simulink model "punto_33"  (R2015a)
settings: Solver=ode45  StartTime=0.0  StopTime=10.0  RelTol=1e-3
values from neighbouring files (symbols this model uses):
  a = [-6 -11 -6;1 0 0;0 1 0]    [punto_1.m]    (also in punto_2.m = [0 1 0;0 0 1;-5 -6 0]; punto_3.m = [0 1 0;0 0 1;-1.244 -0.3956 -3.145]; punto_4.m = [0 1;0 0])
  Aaux = Abb-Ko*Aab    [punto_3.m]    (also in punto_4.m)
  b = [1;0;0]    [punto_1.m]    (also in punto_2.m = [0;0;1]; punto_3.m = [0;0;1.244]; punto_4.m = [0;1])
  Baux = Aaux*Ko+Aba+Ko*Aaa    [punto_3.m]    (also in punto_4.m)
  c = [0 0 10]    [punto_1.m]    (also in punto_2.m = [1 0 0]; punto_3.m = [1 0 0]; punto_4.m = [1 0])
  d = 0    [punto_1.m]    (also in punto_2.m; punto_3.m; punto_4.m)
  F = Bb-(Ko*Ba)    [punto_3.m]    (also in punto_4.m)
  k = place(a,b,p)    [punto_1.m]    (also in punto_2.m = acker(a,b,p); punto_3.m = place(a,b,p1); punto_4.m = place(a,b,prealim))
  Ko = acker(a',c',p)'    [punto_2.m]    (also in punto_3.m = place(Abb',Aab',p)'; punto_4.m = place(Abb',Aab',pobsv)')
settings Model: Creator=Jose Roldan  LastModifiedBy=Jose Roldan

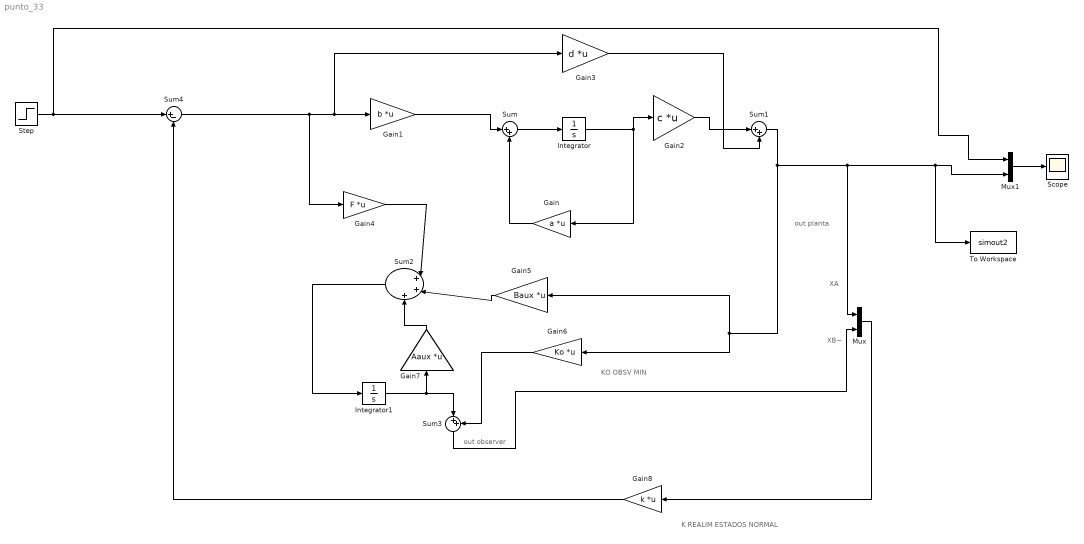
== system punto_33 ==
  note: KO OBSV MIN
  note: K REALIM ESTADOS NORMAL
  note: out planta
  note: out observer
  note: XB~
  note: XA
  Gain : Gain  Gain=a  Multiplication=Matrix(K*u)
  Gain1 : Gain  Gain=b  Multiplication=Matrix(K*u)
  Gain2 : Gain  Gain=c  Multiplication=Matrix(K*u)
  Gain3 : Gain  Gain=d  Multiplication=Matrix(K*u)
  Gain4 : Gain  Gain=F  Multiplication=Matrix(K*u)
  Gain5 : Gain  Gain=Baux  Multiplication=Matrix(K*u)
  Gain6 : Gain  Gain=Ko  Multiplication=Matrix(K*u)
  Gain7 : Gain  Gain=Aaux  Multiplication=Matrix(K*u)
  Gain8 : Gain  Gain=k  Multiplication=Matrix(K*u)
  Integrator : Integrator
  Integrator1 : Integrator
  Mux : Mux  Inputs=2
  Mux1 : Mux  Inputs=2
  Scope : Scope
  Step : Step  SampleTime=0
  Sum : Sum  Inputs=|++
  Sum1 : Sum  Inputs=|++
  Sum2 : Sum  Inputs=|+++
  Sum3 : Sum  Inputs=|++
  Sum4 : Sum  Inputs=|+-
  To Workspace : ToWorkspace  VariableName=simout2  SaveFormat=Timeseries  SampleTime=-1
  wires:
  Gain1/1 -> Sum/1
  Sum/1 -> Integrator/1
  Integrator/1 -> Gain/1, Gain2/1
  Gain2/1 -> Sum1/1
  Gain3/1 -> Sum1/2
  Gain/1 -> Sum/2
  Gain4/1 -> Sum2/1
  Sum2/1 -> Integrator1/1
  Gain7/1 -> Sum2/3
  Integrator1/1 -> Sum3/1, Gain7/1
  Gain6/1 -> Sum3/2
  Sum1/1 -> Gain6/1, Gain5/1, Mux/1, To Workspace/1, Mux1/2
  Gain5/1 -> Sum2/2
  Sum3/1 -> Mux/2
  Mux/1 -> Gain8/1
  Gain8/1 -> Sum4/2
  Sum4/1 -> Gain4/1, Gain3/1, Gain1/1
  Step/1 -> Sum4/1, Mux1/1
  Mux1/1 -> Scope/1
